simulink model "Dynamics"  (R2023a)
settings: Solver=FixedStepAuto  StartTime=0.0  StopTime=inf  FixedStep=0.001  EnableMultiTasking=on
libraries: sharedutil x32, sharedtransform x18, dspmtrx3 x12, matrix_library x6, simulink_extras x1, simulink x1
(part 2 of 6)

== system Dynamics/Subsystem/Z ==
  J(q) : Inport
  dq : Inport  Port=2
  Demux : Demux  Outputs=36
  Mux{,1..11} (12 alike) : Mux  Inputs=3
  Product : Product  Multiplication=Matrix(*)
  v1 : Outport
  v2 : Outport  Port=2
  v3 : Outport  Port=3
  v4 : Outport  Port=4
  v5 : Outport  Port=5
  v6 : Outport  Port=6
  w1 : Outport  Port=7
  w2 : Outport  Port=8
  w3 : Outport  Port=9
  w4 : Outport  Port=10
  w5 : Outport  Port=11
  w6 : Outport  Port=12
  Z : Outport  Port=13
  wires:
  J(q)/1 -> Product/1
  dq/1 -> Product/2
  Product/1 -> Z/1, Demux/1
  Demux/1 -> Mux/1
  Demux/2 -> Mux/2
  Demux/3 -> Mux/3
  Mux/1 -> v1/1
  Demux/4 -> Mux1/1
  Demux/5 -> Mux1/2
  Demux/6 -> Mux1/3
  Mux1/1 -> v2/1
  Mux2/1 -> v3/1
  Demux/7 -> Mux2/1
  Demux/8 -> Mux2/2
  Demux/9 -> Mux2/3
  Mux3/1 -> v4/1
  Demux/10 -> Mux3/1
  Demux/11 -> Mux3/2
  Demux/12 -> Mux3/3
  Mux4/1 -> v5/1
  Demux/14 -> Mux4/2
  Demux/13 -> Mux4/1
  Demux/15 -> Mux4/3
  Mux5/1 -> v6/1
  Demux/17 -> Mux5/2
  Demux/16 -> Mux5/1
  Demux/18 -> Mux5/3
  Mux6/1 -> w1/1
  Demux/19 -> Mux6/1
  Demux/20 -> Mux6/2
  Demux/21 -> Mux6/3
  Mux7/1 -> w2/1
  Demux/22 -> Mux7/1
  Demux/23 -> Mux7/2
  Demux/24 -> Mux7/3
  Mux8/1 -> w3/1
  Demux/25 -> Mux8/1
  Demux/26 -> Mux8/2
  Demux/27 -> Mux8/3
  Mux9/1 -> w4/1
  Demux/28 -> Mux9/1
  Demux/29 -> Mux9/2
  Demux/30 -> Mux9/3
  Mux10/1 -> w5/1
  Demux/31 -> Mux10/1
  Demux/32 -> Mux10/2
  Demux/33 -> Mux10/3
  Mux11/1 -> w6/1
  Demux/34 -> Mux11/1
  Demux/35 -> Mux11/2
  Demux/36 -> Mux11/3

== system Dynamics/Subsystem/tau(t) ==
  g(q) : Inport
  Add : Sum
  Constant : Constant  Value=zeros(5,1)
  Gain : Gain  Gain=0
  Mux : Mux  Inputs=2
  Sine Wave : Sin  SampleTime=0
  tau : Outport
  wires:
  Sine Wave/1 -> Mux/2
  Constant/1 -> Mux/1
  Add/1 -> tau/1
  Mux/1 -> Gain/1
  g(q)/1 -> Add/1
  Gain/1 -> Add/2

== system Dynamics/Subsystem2/Dynamics ==
  M(q) : Inport
  C(q,dq) : Inport  Port=2
  g(q) : Inport  Port=3
  dq : Inport  Port=4
  tau : Inport  Port=5
  q0 : Inport  Port=6
  dq0 : Inport  Port=7
  Add : Sum
  Add1 : Sum
  Gain : Gain  Gain=-1
  "Integrator, Second-Order" : SecondOrderIntegrator  ICSourceX=external  ICSourceDXDT=external
  Interpreted MATLAB Function : MATLABFcn  MATLABFcn=inv  OutputSignalType=real  Output1D=off
  Product : Product  Multiplication=Matrix(*)
  Product1 : Product  Multiplication=Matrix(*)
  q+delta_q : Outport
  dq+delta_dq : Outport  Port=2
  wires:
  C(q,dq)/1 -> Product/1
  dq/1 -> Product/2
  Product/1 -> Add/1
  g(q)/1 -> Add/2
  Add/1 -> Gain/1
  M(q)/1 -> Interpreted MATLAB Function/1
  Interpreted MATLAB Function/1 -> Product1/1
  Gain/1 -> Add1/1
  tau/1 -> Add1/2
  Add1/1 -> Product1/2
  Product1/1 -> "Integrator, Second-Order"/1
  "Integrator, Second-Order"/2 -> dq+delta_dq/1
  "Integrator, Second-Order"/1 -> q+delta_q/1
  q0/1 -> "Integrator, Second-Order"/2
  dq0/1 -> "Integrator, Second-Order"/3

== system Dynamics/Subsystem2/F gen. ==
  M : Inport
  H : Inport  Port=2
  G : Inport  Port=3
  Z : Inport  Port=4
  Add : Sum  Inputs=+++
  Derivative : Derivative
  Product1 : Product  Multiplication=Matrix(*)
  Product2 : Product  Multiplication=Matrix(*)
  F : Outport
  wires:
  Z/1 -> Product1/2, Derivative/1
  Add/1 -> F/1
  G/1 -> Add/3
  Product2/1 -> Add/1
  M/1 -> Product2/1
  Derivative/1 -> Product2/2
  Product1/1 -> Add/2
  H/1 -> Product1/1

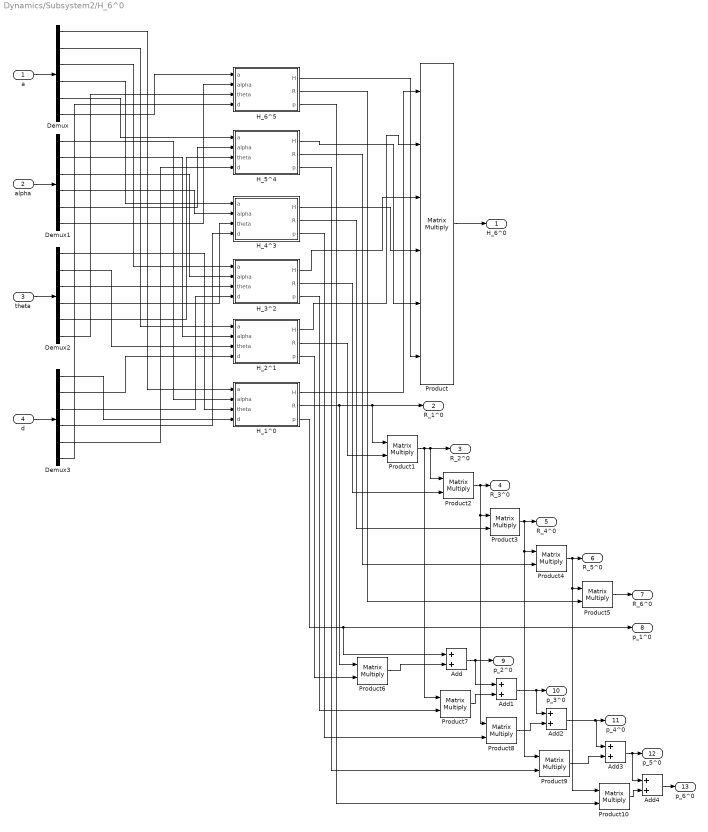
== system Dynamics/Subsystem2/H_6^0 ==
  a : Inport
  alpha : Inport  Port=2
  theta : Inport  Port=3
  d : Inport  Port=4
  Add{,1..4} (5 alike) : Sum
  Demux{,1..3} (4 alike) : Demux  Outputs=6
  H_1^0 : Subsystem
  H_2^1 : Subsystem
  H_3^2 : Subsystem
  H_4^3 : Subsystem
  H_5^4 : Subsystem
  H_6^5 : Subsystem
  Product : Product  Inputs=6  Multiplication=Matrix(*)
  Product{1..10} (10 alike) : Product  Multiplication=Matrix(*)
  H_6^0 : Outport
  R_1^0 : Outport  Port=2
  R_2^0 : Outport  Port=3
  R_3^0 : Outport  Port=4
  R_4^0 : Outport  Port=5
  R_5^0 : Outport  Port=6
  R_6^0 : Outport  Port=7
  p_1^0 : Outport  Port=8
  p_2^0 : Outport  Port=9
  p_3^0 : Outport  Port=10
  p_4^0 : Outport  Port=11
  p_5^0 : Outport  Port=12
  p_6^0 : Outport  Port=13
  wires:
  H_6^5/1(H) -> Product/6
  H_5^4/1(H) -> Product/5
  H_2^1/1(H) -> Product/2
  H_1^0/1(H) -> Product/1
  Product/1 -> H_6^0/1
  a/1 -> Demux/1
  d/1 -> Demux3/1
  H_4^3/1(H) -> Product/4
  H_3^2/1(H) -> Product/3
  Product1/1 -> Product7/1, Product2/1, R_2^0/1
  H_2^1/2(R) -> Product1/2
  Product2/1 -> Product8/1, Product3/1, R_3^0/1
  Product3/1 -> Product9/1, Product4/1, R_4^0/1
  Product4/1 -> Product10/1, Product5/1, R_5^0/1
  Product5/1 -> R_6^0/1
  Add/1 -> Add1/1, p_2^0/1
  theta/1 -> Demux2/1
  alpha/1 -> Demux1/1
  Demux/1 -> H_1^0/1(a)
  Demux/6 -> H_6^5/1(a)
  Demux/5 -> H_5^4/1(a)
  Demux/4 -> H_4^3/1(a)
  Demux/3 -> H_3^2/1(a)
  Demux/2 -> H_2^1/1(a)
  Demux1/6 -> H_6^5/2(alpha)
  Demux1/5 -> H_5^4/2(alpha)
  Demux1/4 -> H_4^3/2(alpha)
  Demux1/3 -> H_3^2/2(alpha)
  Demux1/2 -> H_2^1/2(alpha)
  Demux1/1 -> H_1^0/2(alpha)
  Demux2/6 -> H_6^5/3(theta)
  Demux2/5 -> H_5^4/3(theta)
  Demux2/4 -> H_4^3/3(theta)
  Demux2/3 -> H_3^2/3(theta)
  Demux2/2 -> H_2^1/3(theta)
  Demux2/1 -> H_1^0/3(theta)
  Demux3/1 -> H_1^0/4(d)
  Demux3/2 -> H_2^1/4(d)
  Demux3/3 -> H_3^2/4(d)
  Demux3/4 -> H_4^3/4(d)
  Demux3/5 -> H_5^4/4(d)
  Demux3/6 -> H_6^5/4(d)
  H_3^2/2(R) -> Product2/2
  H_4^3/2(R) -> Product3/2
  H_5^4/2(R) -> Product4/2
  H_6^5/2(R) -> Product5/2
  H_1^0/3(p) -> Add/1, p_1^0/1
  H_2^1/3(p) -> Product6/2
  Add1/1 -> Add2/1, p_3^0/1
  H_3^2/3(p) -> Product7/2
  H_4^3/3(p) -> Product8/2
  Add2/1 -> Add3/1, p_4^0/1
  H_5^4/3(p) -> Product9/2
  Add3/1 -> Add4/1, p_5^0/1
  H_6^5/3(p) -> Product10/2
  Add4/1 -> p_6^0/1
  H_1^0/2(R) -> R_1^0/1, Product1/1, Product6/1
  Product6/1 -> Add/2
  Product7/1 -> Add1/2
  Product8/1 -> Add2/2
  Product9/1 -> Add3/2
  Product10/1 -> Add4/2

== system Dynamics/Subsystem2/Jacobian ==
  R_1^0 : Inport
  R_2^0 : Inport  Port=2
  R_3^0 : Inport  Port=3
  R_4^0 : Inport  Port=4
  R_5^0 : Inport  Port=5
  R_6^0 : Inport  Port=6
  p_1^0 : Inport  Port=7
  p_2^0 : Inport  Port=8
  p_3^0 : Inport  Port=9
  p_4^0 : Inport  Port=10
  p_5^0 : Inport  Port=11
  p_6^0 : Inport  Port=12
  type1 : Inport  Port=13
  type2 : Inport  Port=14
  type3 : Inport  Port=15
  type4 : Inport  Port=16
  type5 : Inport  Port=17
  type6 : Inport  Port=18
  J(q) gen. : Subsystem
  J_v : Subsystem
  J_w : Subsystem
  Vector Concatenate : Concatenate  Mode=Multidimensional array
  J : Outport
  J(q) : Outport  Port=2
  wires:
  R_1^0/1 -> J_v/1(R_1^0), J_w/1(R_1^0), J(q) gen./1(R_1^0)
  p_1^0/1 -> J_v/7(p_1^0), J(q) gen./7(p_1^0)
  p_2^0/1 -> J_v/8(p_2^0), J(q) gen./8(p_2^0)
  p_3^0/1 -> J_v/9(p_3^0), J(q) gen./9(p_3^0)
  p_4^0/1 -> J_v/10(p_4^0), J(q) gen./10(p_4^0)
  p_5^0/1 -> J_v/11(p_5^0), J(q) gen./11(p_5^0)
  R_2^0/1 -> J_v/2(R_2^0), J_w/2(R_2^0), J(q) gen./2(R_2^0)
  R_3^0/1 -> J_v/3(R_3^0), J_w/3(R_3^0), J(q) gen./3(R_3^0)
  R_4^0/1 -> J_v/4(R_4^0), J_w/4(R_4^0), J(q) gen./4(R_4^0)
  R_5^0/1 -> J_v/5(R_5^0), J_w/5(R_5^0), J(q) gen./5(R_5^0)
  type1/1 -> J_w/7(type1), J_v/13(type1), J(q) gen./12(type1)
  type2/1 -> J_w/8(type2), J(q) gen./13(type2), J_v/14(type2)
  type3/1 -> J_w/9(type3), J(q) gen./14(type3), J_v/15(type3)
  type4/1 -> J_w/10(type4), J(q) gen./15(type4), J_v/16(type4)
  type5/1 -> J_w/11(type5), J_v/17(type5)
  type6/1 -> J_w/12(type6), J_v/18(type6)
  p_6^0/1 -> J_v/12(p_6^0)
  J_v/1(J_v) -> J(q) gen./16(J_v_6(q)), Vector Concatenate/1
  J_w/1(EF J_w) -> Vector Concatenate/2
  Vector Concatenate/1 -> J/1
  J(q) gen./1(J(q)) -> J(q)/1
  J_w/2(J_w1) -> J(q) gen./17(J_w1)
  J_w/3(J_w2) -> J(q) gen./18(J_w2)
  J_w/4(J_w3) -> J(q) gen./19(J_w3)
  J_w/5(J_w4) -> J(q) gen./20(J_w4)
  J_w/6(J_w5) -> J(q) gen./21(J_w5)
  J_w/7(J_w6) -> J(q) gen./22(J_w6)
  R_6^0/1 -> J_v/6(R_6^0), J_w/6(R_6^0), J(q) gen./6(R_6^0)

== system Dynamics/Subsystem2/M(q),C(q,dq),g(q) ==
  m : Inport
  J(q) : Inport  Port=2
  I1 : Inport  Port=3
  I2 : Inport  Port=4
  I3 : Inport  Port=5
  I4 : Inport  Port=6
  I5 : Inport  Port=7
  I6 : Inport  Port=8
  w1 : Inport  Port=9
  w2 : Inport  Port=10
  w3 : Inport  Port=11
  w4 : Inport  Port=12
  w5 : Inport  Port=13
  w6 : Inport  Port=14
  Add : Sum
  G gen : Subsystem
  Interpreted MATLAB Function : MATLABFcn  MATLABFcn=transpose  OutputSignalType=real  Output1D=off
  M,H : Subsystem
  Product{,1..3} (4 alike) : Product  Multiplication=Matrix(*)
  Product4 : Product  Inputs=3  Multiplication=Matrix(*)
  dJ : Derivative
  g(q) : Outport
  C(q,dq) : Outport  Port=2
  M(q) : Outport  Port=3
  M : Outport  Port=4
  H : Outport  Port=5
  G : Outport  Port=6
  wires:
  J(q)/1 -> Interpreted MATLAB Function/1, Product4/3, Product2/2, dJ/1
  Interpreted MATLAB Function/1 -> Product4/1, Product3/1, Product/1
  Product/1 -> g(q)/1
  m/1 -> G gen/1(m), M,H/1(m)
  I1/1 -> M,H/2(I1)
  I2/1 -> M,H/3(I2)
  I3/1 -> M,H/4(I3)
  I4/1 -> M,H/5(I4)
  I5/1 -> M,H/6(I5)
  I6/1 -> M,H/7(I6)
  w1/1 -> M,H/8(w1)
  w2/1 -> M,H/9(w2)
  w3/1 -> M,H/10(w3)
  w4/1 -> M,H/11(w4)
  w5/1 -> M,H/12(w5)
  w6/1 -> M,H/13(w6)
  M,H/1(M) -> Product1/1, M/1, Product4/2
  dJ/1 -> Product1/2
  M,H/2(H) -> H/1, Product2/1
  Product1/1 -> Add/1
  Product2/1 -> Add/2
  Add/1 -> Product3/2
  Product3/1 -> C(q,dq)/1
  Product4/1 -> M(q)/1
  G gen/1(G) -> G/1, Product/2

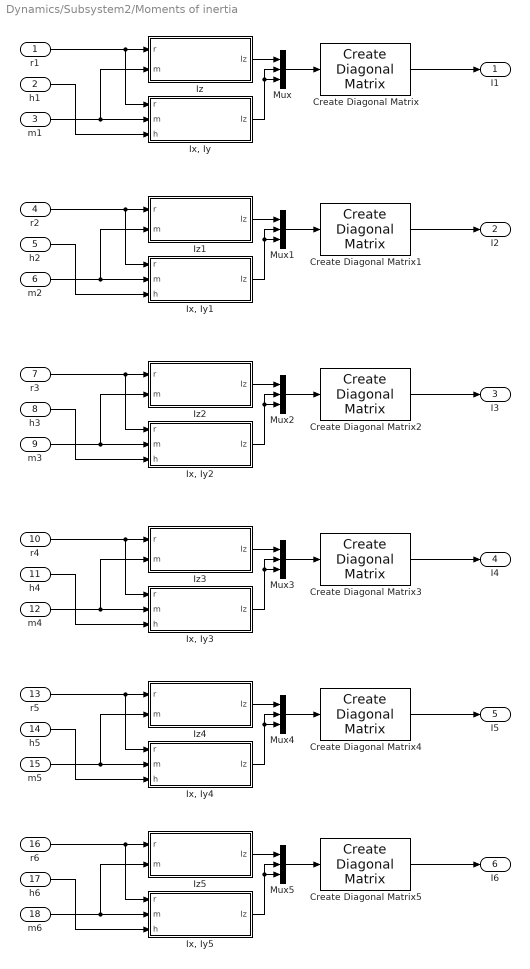
== system Dynamics/Subsystem2/Moments of inertia ==
  r1 : Inport
  h1 : Inport  Port=2
  m1 : Inport  Port=3
  r2 : Inport  Port=4
  h2 : Inport  Port=5
  m2 : Inport  Port=6
  r3 : Inport  Port=7
  h3 : Inport  Port=8
  m3 : Inport  Port=9
  r4 : Inport  Port=10
  h4 : Inport  Port=11
  m4 : Inport  Port=12
  r5 : Inport  Port=13
  h5 : Inport  Port=14
  m5 : Inport  Port=15
  r6 : Inport  Port=16
  h6 : Inport  Port=17
  m6 : Inport  Port=18
  Create Diagonal Matrix{,1..5} (6 alike) : matrix_library/Create Diagonal Matrix
  "Ix, Iy" : Subsystem
  "Ix, Iy1" : Subsystem
  "Ix, Iy2" : Subsystem
  "Ix, Iy3" : Subsystem
  "Ix, Iy4" : Subsystem
  "Ix, Iy5" : Subsystem
  Iz : Subsystem
  Iz1 : Subsystem
  Iz2 : Subsystem
  Iz3 : Subsystem
  Iz4 : Subsystem
  Iz5 : Subsystem
  Mux{,1..5} (6 alike) : Mux  Inputs=3
  I1 : Outport
  I2 : Outport  Port=2
  I3 : Outport  Port=3
  I4 : Outport  Port=4
  I5 : Outport  Port=5
  I6 : Outport  Port=6
  wires:
  r1/1 -> "Ix, Iy"/1(r), Iz/1(r)
  m1/1 -> "Ix, Iy"/2(m), Iz/2(m)
  h1/1 -> "Ix, Iy"/3(h)
  Mux/1 -> Create Diagonal Matrix/1
  Iz/1(Iz) -> Mux/1
  "Ix, Iy"/1(Iz) -> Mux/3, Mux/2
  Create Diagonal Matrix/1 -> I1/1
  r2/1 -> "Ix, Iy1"/1(r), Iz1/1(r)
  m2/1 -> "Ix, Iy1"/2(m), Iz1/2(m)
  h2/1 -> "Ix, Iy1"/3(h)
  Mux1/1 -> Create Diagonal Matrix1/1
  Iz1/1(Iz) -> Mux1/1
  "Ix, Iy1"/1(Iz) -> Mux1/3, Mux1/2
  Create Diagonal Matrix1/1 -> I2/1
  r3/1 -> "Ix, Iy2"/1(r), Iz2/1(r)
  m3/1 -> "Ix, Iy2"/2(m), Iz2/2(m)
  h3/1 -> "Ix, Iy2"/3(h)
  Mux2/1 -> Create Diagonal Matrix2/1
  Iz2/1(Iz) -> Mux2/1
  "Ix, Iy2"/1(Iz) -> Mux2/3, Mux2/2
  Create Diagonal Matrix2/1 -> I3/1
  r4/1 -> "Ix, Iy3"/1(r), Iz3/1(r)
  m4/1 -> "Ix, Iy3"/2(m), Iz3/2(m)
  h4/1 -> "Ix, Iy3"/3(h)
  Mux3/1 -> Create Diagonal Matrix3/1
  Iz3/1(Iz) -> Mux3/1
  "Ix, Iy3"/1(Iz) -> Mux3/3, Mux3/2
  Create Diagonal Matrix3/1 -> I4/1
  r5/1 -> "Ix, Iy4"/1(r), Iz4/1(r)
  m5/1 -> "Ix, Iy4"/2(m), Iz4/2(m)
  h5/1 -> "Ix, Iy4"/3(h)
  Mux4/1 -> Create Diagonal Matrix4/1
  Iz4/1(Iz) -> Mux4/1
  "Ix, Iy4"/1(Iz) -> Mux4/3, Mux4/2
  Create Diagonal Matrix4/1 -> I5/1
  r6/1 -> "Ix, Iy5"/1(r), Iz5/1(r)
  m6/1 -> "Ix, Iy5"/2(m), Iz5/2(m)
  h6/1 -> "Ix, Iy5"/3(h)
  Mux5/1 -> Create Diagonal Matrix5/1
  Iz5/1(Iz) -> Mux5/1
  "Ix, Iy5"/1(Iz) -> Mux5/3, Mux5/2
  Create Diagonal Matrix5/1 -> I6/1

== system Dynamics/Subsystem2/Slotine ==
  g(q) : Inport
  C(q,dq) : Inport  Port=2
  M(q) : Inport  Port=3
  q_d : Inport  Port=4
  dq_d : Inport  Port=5
  ddq_d : Inport  Port=6
  q : Inport  Port=7
  dq : Inport  Port=8
  Lambda : Inport  Port=9
  K : Inport  Port=10
  S-gen : Subsystem
  V-gen : Subsystem
  dV-gen : Subsystem
  dq_tilde : Sum  Inputs=-+
  q_tilde : Sum  Inputs=-+
  tau-gen : Subsystem
  tau : Outport
  wires:
  q_d/1 -> q_tilde/1
  q/1 -> q_tilde/2
  dq_d/1 -> V-gen/2(dq_d), dq_tilde/1
  dq/1 -> S-gen/1(dq), dq_tilde/2
  ddq_d/1 -> dV-gen/2(ddq_d)
  q_tilde/1 -> V-gen/1(q_tilde)
  Lambda/1 -> dV-gen/3(Gamma), V-gen/3(Gamma)
  dq_tilde/1 -> dV-gen/1(dq_tilde)
  V-gen/1(V) -> tau-gen/4(V), S-gen/2(V)
  M(q)/1 -> tau-gen/1(M)
  C(q,dq)/1 -> tau-gen/2(C)
  g(q)/1 -> tau-gen/3(g)
  dV-gen/1(dV) -> tau-gen/5(dV)
  S-gen/1(S) -> tau-gen/6(S)
  K/1 -> tau-gen/7(K)
  tau-gen/1(tau) -> tau/1

== system Dynamics/Subsystem2/Z ==
  J(q) : Inport
  dq : Inport  Port=2
  Demux : Demux  Outputs=36
  Mux{,1..11} (12 alike) : Mux  Inputs=3
  Product : Product  Multiplication=Matrix(*)
  v1 : Outport
  v2 : Outport  Port=2
  v3 : Outport  Port=3
  v4 : Outport  Port=4
  v5 : Outport  Port=5
  v6 : Outport  Port=6
  w1 : Outport  Port=7
  w2 : Outport  Port=8
  w3 : Outport  Port=9
  w4 : Outport  Port=10
  w5 : Outport  Port=11
  w6 : Outport  Port=12
  Z : Outport  Port=13
  wires:
  J(q)/1 -> Product/1
  dq/1 -> Product/2
  Product/1 -> Z/1, Demux/1
  Demux/1 -> Mux/1
  Demux/2 -> Mux/2
  Demux/3 -> Mux/3
  Mux/1 -> v1/1
  Demux/4 -> Mux1/1
  Demux/5 -> Mux1/2
  Demux/6 -> Mux1/3
  Mux1/1 -> v2/1
  Mux2/1 -> v3/1
  Demux/7 -> Mux2/1
  Demux/8 -> Mux2/2
  Demux/9 -> Mux2/3
  Mux3/1 -> v4/1
  Demux/10 -> Mux3/1
  Demux/11 -> Mux3/2
  Demux/12 -> Mux3/3
  Mux4/1 -> v5/1
  Demux/14 -> Mux4/2
  Demux/13 -> Mux4/1
  Demux/15 -> Mux4/3
  Mux5/1 -> v6/1
  Demux/17 -> Mux5/2
  Demux/16 -> Mux5/1
  Demux/18 -> Mux5/3
  Mux6/1 -> w1/1
  Demux/19 -> Mux6/1
  Demux/20 -> Mux6/2
  Demux/21 -> Mux6/3
  Mux7/1 -> w2/1
  Demux/22 -> Mux7/1
  Demux/23 -> Mux7/2
  Demux/24 -> Mux7/3
  Mux8/1 -> w3/1
  Demux/25 -> Mux8/1
  Demux/26 -> Mux8/2
  Demux/27 -> Mux8/3
  Mux9/1 -> w4/1
  Demux/28 -> Mux9/1
  Demux/29 -> Mux9/2
  Demux/30 -> Mux9/3
  Mux10/1 -> w5/1
  Demux/31 -> Mux10/1
  Demux/32 -> Mux10/2
  Demux/33 -> Mux10/3
  Mux11/1 -> w6/1
  Demux/34 -> Mux11/1
  Demux/35 -> Mux11/2
  Demux/36 -> Mux11/3

== system Dynamics/Subsystem2/tau(t) ==
  g(q) : Inport
  Add : Sum
  Constant : Constant  Value=zeros(5,1)
  Gain : Gain  Gain=0
  Mux : Mux  Inputs=2
  Sine Wave : Sin  SampleTime=0
  tau : Outport
  wires:
  Sine Wave/1 -> Mux/2
  Constant/1 -> Mux/1
  Add/1 -> tau/1
  Mux/1 -> Gain/1
  g(q)/1 -> Add/1
  Gain/1 -> Add/2

== system Dynamics/DYNAMIC/H_6^0/H_1^0 ==
  a : Inport
  alpha : Inport  Port=2
  theta : Inport  Port=3
  d : Inport  Port=4
  Gain1 : Gain  Gain=-1
  Gain2 : Gain  Gain=-1
  MATLAB Function : MATLAB Function  TreatAsAtomicUnit=on
  Mux : Mux  Inputs=3
  Mux1 : Mux  Inputs=3
  Product : Product
  Product1 : Product
  Rotation Angles to Direction Cosine Matrix : sharedtransform/Rotation Angles to Direction Cosine Matrix  rotationOrder=ZXY  aMode=aMode
  Trigonometric Function : Trigonometry  Operator=cos
  Trigonometric Function1 : Trigonometry
  Zero : Constant  Value=0
  H : Outport
  R : Outport  Port=2
  p : Outport  Port=3
  wires:
  Mux/1 -> Rotation Angles to Direction Cosine Matrix/1
  alpha/1 -> Gain1/1
  Zero/1 -> Mux/3
  Rotation Angles to Direction Cosine Matrix/1 -> MATLAB Function/1(R), R/1
  Mux1/1 -> MATLAB Function/2(p), p/1
  Trigonometric Function/1 -> Product/1
  Trigonometric Function1/1 -> Product1/1
  Product/1 -> Mux1/1
  Product1/1 -> Mux1/2
  a/1 -> Product/2, Product1/2
  MATLAB Function/1(H) -> H/1
  Gain1/1 -> Mux/1
  Gain2/1 -> Mux/2
  theta/1 -> Trigonometric Function1/1, Trigonometric Function/1, Gain2/1
  d/1 -> Mux1/3

== system Dynamics/DYNAMIC/H_6^0/H_2^1 ==
  a : Inport
  alpha : Inport  Port=2
  theta : Inport  Port=3
  d : Inport  Port=4
  Gain1 : Gain  Gain=-1
  Gain2 : Gain  Gain=-1
  MATLAB Function : MATLAB Function  TreatAsAtomicUnit=on
  Mux : Mux  Inputs=3
  Mux1 : Mux  Inputs=3
  Product : Product
  Product1 : Product
  Rotation Angles to Direction Cosine Matrix : sharedtransform/Rotation Angles to Direction Cosine Matrix  rotationOrder=ZXY  aMode=aMode
  Trigonometric Function : Trigonometry  Operator=cos
  Trigonometric Function1 : Trigonometry
  Zero : Constant  Value=0
  H : Outport
  R : Outport  Port=2
  p : Outport  Port=3
  wires:
  Mux/1 -> Rotation Angles to Direction Cosine Matrix/1
  alpha/1 -> Gain1/1
  Zero/1 -> Mux/3
  Rotation Angles to Direction Cosine Matrix/1 -> MATLAB Function/1(R), R/1
  Mux1/1 -> MATLAB Function/2(p), p/1
  Trigonometric Function/1 -> Product/1
  Trigonometric Function1/1 -> Product1/1
  Product/1 -> Mux1/1
  Product1/1 -> Mux1/2
  a/1 -> Product/2, Product1/2
  MATLAB Function/1(H) -> H/1
  Gain1/1 -> Mux/1
  Gain2/1 -> Mux/2
  theta/1 -> Trigonometric Function1/1, Trigonometric Function/1, Gain2/1
  d/1 -> Mux1/3

== system Dynamics/DYNAMIC/H_6^0/H_3^2 ==
  a : Inport
  alpha : Inport  Port=2
  theta : Inport  Port=3
  d : Inport  Port=4
  Gain1 : Gain  Gain=-1
  Gain2 : Gain  Gain=-1
  MATLAB Function : MATLAB Function  TreatAsAtomicUnit=on
  Mux : Mux  Inputs=3
  Mux1 : Mux  Inputs=3
  Product : Product
  Product1 : Product
  Rotation Angles to Direction Cosine Matrix : sharedtransform/Rotation Angles to Direction Cosine Matrix  rotationOrder=ZXY  aMode=aMode
  Trigonometric Function : Trigonometry  Operator=cos
  Trigonometric Function1 : Trigonometry
  Zero : Constant  Value=0
  H : Outport
  R : Outport  Port=2
  p : Outport  Port=3
  wires:
  Mux/1 -> Rotation Angles to Direction Cosine Matrix/1
  alpha/1 -> Gain1/1
  Zero/1 -> Mux/3
  Rotation Angles to Direction Cosine Matrix/1 -> MATLAB Function/1(R), R/1
  Mux1/1 -> MATLAB Function/2(p), p/1
  Trigonometric Function/1 -> Product/1
  Trigonometric Function1/1 -> Product1/1
  Product/1 -> Mux1/1
  Product1/1 -> Mux1/2
  a/1 -> Product/2, Product1/2
  MATLAB Function/1(H) -> H/1
  Gain1/1 -> Mux/1
  Gain2/1 -> Mux/2
  theta/1 -> Trigonometric Function1/1, Trigonometric Function/1, Gain2/1
  d/1 -> Mux1/3

== system Dynamics/DYNAMIC/H_6^0/H_4^3 ==
  a : Inport
  alpha : Inport  Port=2
  theta : Inport  Port=3
  d : Inport  Port=4
  Gain1 : Gain  Gain=-1
  Gain2 : Gain  Gain=-1
  MATLAB Function : MATLAB Function  TreatAsAtomicUnit=on
  Mux : Mux  Inputs=3
  Mux1 : Mux  Inputs=3
  Product : Product
  Product1 : Product
  Rotation Angles to Direction Cosine Matrix : sharedtransform/Rotation Angles to Direction Cosine Matrix  rotationOrder=ZXY  aMode=aMode
  Trigonometric Function : Trigonometry  Operator=cos
  Trigonometric Function1 : Trigonometry
  Zero : Constant  Value=0
  H : Outport
  R : Outport  Port=2
  p : Outport  Port=3
  wires:
  Mux/1 -> Rotation Angles to Direction Cosine Matrix/1
  alpha/1 -> Gain1/1
  Zero/1 -> Mux/3
  Rotation Angles to Direction Cosine Matrix/1 -> MATLAB Function/1(R), R/1
  Mux1/1 -> MATLAB Function/2(p), p/1
  Trigonometric Function/1 -> Product/1
  Trigonometric Function1/1 -> Product1/1
  Product/1 -> Mux1/1
  Product1/1 -> Mux1/2
  a/1 -> Product/2, Product1/2
  MATLAB Function/1(H) -> H/1
  Gain1/1 -> Mux/1
  Gain2/1 -> Mux/2
  theta/1 -> Trigonometric Function1/1, Trigonometric Function/1, Gain2/1
  d/1 -> Mux1/3

== system Dynamics/DYNAMIC/H_6^0/H_5^4 ==
  a : Inport
  alpha : Inport  Port=2
  theta : Inport  Port=3
  d : Inport  Port=4
  Gain1 : Gain  Gain=-1
  Gain2 : Gain  Gain=-1
  MATLAB Function : MATLAB Function  TreatAsAtomicUnit=on
  Mux : Mux  Inputs=3
  Mux1 : Mux  Inputs=3
  Product : Product
  Product1 : Product
  Rotation Angles to Direction Cosine Matrix : sharedtransform/Rotation Angles to Direction Cosine Matrix  rotationOrder=ZXY  aMode=aMode
  Trigonometric Function : Trigonometry  Operator=cos
  Trigonometric Function1 : Trigonometry
  Zero : Constant  Value=0
  H : Outport
  R : Outport  Port=2
  p : Outport  Port=3
  wires:
  Mux/1 -> Rotation Angles to Direction Cosine Matrix/1
  alpha/1 -> Gain1/1
  Zero/1 -> Mux/3
  Rotation Angles to Direction Cosine Matrix/1 -> MATLAB Function/1(R), R/1
  Mux1/1 -> MATLAB Function/2(p), p/1
  Trigonometric Function/1 -> Product/1
  Trigonometric Function1/1 -> Product1/1
  Product/1 -> Mux1/1
  Product1/1 -> Mux1/2
  a/1 -> Product/2, Product1/2
  MATLAB Function/1(H) -> H/1
  Gain1/1 -> Mux/1
  Gain2/1 -> Mux/2
  theta/1 -> Trigonometric Function1/1, Trigonometric Function/1, Gain2/1
  d/1 -> Mux1/3

== system Dynamics/DYNAMIC/H_6^0/H_6^5 ==
  a : Inport
  alpha : Inport  Port=2
  theta : Inport  Port=3
  d : Inport  Port=4
  Gain1 : Gain  Gain=-1
  Gain2 : Gain  Gain=-1
  MATLAB Function : MATLAB Function  TreatAsAtomicUnit=on
  Mux : Mux  Inputs=3
  Mux1 : Mux  Inputs=3
  Product : Product
  Product1 : Product
  Rotation Angles to Direction Cosine Matrix : sharedtransform/Rotation Angles to Direction Cosine Matrix  rotationOrder=ZXY  aMode=aMode
  Trigonometric Function : Trigonometry  Operator=cos
  Trigonometric Function1 : Trigonometry
  Zero : Constant  Value=0
  H : Outport
  R : Outport  Port=2
  p : Outport  Port=3
  wires:
  Mux/1 -> Rotation Angles to Direction Cosine Matrix/1
  alpha/1 -> Gain1/1
  Zero/1 -> Mux/3
  Rotation Angles to Direction Cosine Matrix/1 -> MATLAB Function/1(R), R/1
  Mux1/1 -> MATLAB Function/2(p), p/1
  Trigonometric Function/1 -> Product/1
  Trigonometric Function1/1 -> Product1/1
  Product/1 -> Mux1/1
  Product1/1 -> Mux1/2
  a/1 -> Product/2, Product1/2
  MATLAB Function/1(H) -> H/1
  Gain1/1 -> Mux/1
  Gain2/1 -> Mux/2
  theta/1 -> Trigonometric Function1/1, Trigonometric Function/1, Gain2/1
  d/1 -> Mux1/3

== system Dynamics/DYNAMIC/Jacobian/J(q) gen. ==
  R_1^0 : Inport
  R_2^0 : Inport  Port=2
  R_3^0 : Inport  Port=3
  R_4^0 : Inport  Port=4
  R_5^0 : Inport  Port=5
  R_6^0 : Inport  Port=6
  p_1^0 : Inport  Port=7
  p_2^0 : Inport  Port=8
  p_3^0 : Inport  Port=9
  p_4^0 : Inport  Port=10
  p_5^0 : Inport  Port=11
  type1 : Inport  Port=12
  type2 : Inport  Port=13
  type3 : Inport  Port=14
  type4 : Inport  Port=15
  J_v_6(q) : Inport  Port=16
  J_w1 : Inport  Port=17
  J_w2 : Inport  Port=18
  J_w3 : Inport  Port=19
  J_w4 : Inport  Port=20
  J_w5 : Inport  Port=21
  J_w6 : Inport  Port=22
  J_v_1(q) : Subsystem
  J_v_2(q) : Subsystem
  J_v_3(q) : Subsystem
  J_v_4(q) : Subsystem
  J_v_5(q) : Subsystem
  MATLAB Function : MATLAB Function  TreatAsAtomicUnit=on
  J(q) : Outport
  wires:
  MATLAB Function/1(J_q) -> J(q)/1
  J_v_6(q)/1 -> MATLAB Function/12(J_v6)
  J_w1/1 -> MATLAB Function/1(J_w1)
  J_w2/1 -> MATLAB Function/2(J_w2)
  J_w3/1 -> MATLAB Function/3(J_w3)
  J_w4/1 -> MATLAB Function/4(J_w4)
  J_w5/1 -> MATLAB Function/5(J_w5)
  J_w6/1 -> MATLAB Function/6(J_w6)
  J_v_1(q)/1(J_v_1(q)) -> MATLAB Function/7(J_v1)
  J_v_2(q)/1(J_v_2(q)) -> MATLAB Function/8(J_v2)
  J_v_3(q)/1(J_v_3(q)) -> MATLAB Function/9(J_v3)
  J_v_4(q)/1(J_v_4(q)) -> MATLAB Function/10(J_v4)
  J_v_5(q)/1(J_v_5(q)) -> MATLAB Function/11(J_v5)
  R_5^0/1 -> MATLAB Function/17(R5)
  R_6^0/1 -> MATLAB Function/18(R6)
  R_1^0/1 -> MATLAB Function/13(R1), J_v_5(q)/1(R_1^0), J_v_4(q)/1(R_1^0), J_v_3(q)/1(R_1^0), J_v_2(q)/1(R_1^0)
  R_2^0/1 -> MATLAB Function/14(R2), J_v_5(q)/2(R_2^0), J_v_4(q)/2(R_2^0), J_v_3(q)/2(R_2^0)
  R_3^0/1 -> J_v_4(q)/3(R_3^0), MATLAB Function/15(R3), J_v_5(q)/3(R_3^0)
  R_4^0/1 -> MATLAB Function/16(R4), J_v_5(q)/4(R_4^0)
  p_1^0/1 -> J_v_5(q)/5(p_1^0), J_v_4(q)/4(p_1^0), J_v_3(q)/3(p_1^0), J_v_2(q)/2(p_1^0)
  p_2^0/1 -> J_v_5(q)/6(p_2^0), J_v_4(q)/5(p_2^0), J_v_3(q)/4(p_2^0), J_v_2(q)/3(p_2^0)
  p_3^0/1 -> J_v_3(q)/5(p_3^0), J_v_5(q)/7(p_3^0), J_v_4(q)/6(p_3^0)
  p_4^0/1 -> J_v_5(q)/8(p_4^0), J_v_4(q)/7(p_4^0)
  p_5^0/1 -> J_v_5(q)/9(p_5^0)
  type1/1 -> J_v_5(q)/10(type1), J_v_4(q)/8(type1), J_v_3(q)/6(type1), J_v_2(q)/4(type1)
  type2/1 -> J_v_5(q)/11(type2), J_v_4(q)/9(type2), J_v_3(q)/7(type2)
  type3/1 -> J_v_5(q)/12(type3), J_v_4(q)/10(type3)
  type4/1 -> J_v_5(q)/13(type4)

== system Dynamics/DYNAMIC/Jacobian/J_v ==
  R_1^0 : Inport
  R_2^0 : Inport  Port=2
  R_3^0 : Inport  Port=3
  R_4^0 : Inport  Port=4
  R_5^0 : Inport  Port=5
  R_6^0 : Inport  Port=6
  p_1^0 : Inport  Port=7
  p_2^0 : Inport  Port=8
  p_3^0 : Inport  Port=9
  p_4^0 : Inport  Port=10
  p_5^0 : Inport  Port=11
  p_6^0 : Inport  Port=12
  type1 : Inport  Port=13
  type2 : Inport  Port=14
  type3 : Inport  Port=15
  type4 : Inport  Port=16
  type5 : Inport  Port=17
  type6 : Inport  Port=18
  J_v_1 : Subsystem
  J_v_2 : Subsystem
  J_v_3 : Subsystem
  J_v_4 : Subsystem
  J_v_5 : Subsystem
  J_v_6 : Subsystem
  v2M_1 : MATLAB Function  TreatAsAtomicUnit=on
  v2M_2 : MATLAB Function  TreatAsAtomicUnit=on
  v2M_3 : MATLAB Function  TreatAsAtomicUnit=on
  v2M_4 : MATLAB Function  TreatAsAtomicUnit=on
  v2M_5 : MATLAB Function  TreatAsAtomicUnit=on
  J_v : Outport
  wires:
  R_1^0/1 -> J_v_1/1(R)
  J_v_1/1(J_v) -> v2M_1/1(v1)
  v2M_1/1(M) -> v2M_2/1(v1)
  v2M_2/1(M) -> v2M_3/1(v1)
  v2M_3/1(M) -> v2M_4/1(v1)
  v2M_4/1(M) -> v2M_5/1(v1)
  v2M_5/1(M) -> J_v/1
  J_v_2/1(J_v) -> v2M_1/2(v2)
  J_v_3/1(J_v) -> v2M_2/2(v2)
  J_v_4/1(J_v) -> v2M_3/2(v2)
  J_v_5/1(J_v) -> v2M_4/2(v2)
  J_v_6/1(J_v) -> v2M_5/2(v2)
  R_2^0/1 -> J_v_2/1(R)
  R_3^0/1 -> J_v_3/1(R)
  R_4^0/1 -> J_v_4/1(R)
  R_5^0/1 -> J_v_5/1(R)
  R_6^0/1 -> J_v_6/1(R)
  p_1^0/1 -> J_v_1/2(p)
  p_2^0/1 -> J_v_2/2(p)
  p_3^0/1 -> J_v_3/2(p)
  p_4^0/1 -> J_v_4/2(p)
  p_5^0/1 -> J_v_5/2(p)
  type2/1 -> J_v_2/4(type)
  type1/1 -> J_v_1/4(type)
  type3/1 -> J_v_3/4(type)
  type4/1 -> J_v_4/4(type)
  type5/1 -> J_v_5/4(type)
  type6/1 -> J_v_6/4(type)
  p_6^0/1 -> J_v_6/2(p), J_v_1/3(pn), J_v_2/3(pn), J_v_3/3(pn), J_v_4/3(pn), J_v_5/3(pn), J_v_6/3(pn)

== system Dynamics/DYNAMIC/Jacobian/J_w ==
  R_1^0 : Inport
  R_2^0 : Inport  Port=2
  R_3^0 : Inport  Port=3
  R_4^0 : Inport  Port=4
  R_5^0 : Inport  Port=5
  R_6^0 : Inport  Port=6
  type1 : Inport  Port=7
  type2 : Inport  Port=8
  type3 : Inport  Port=9
  type4 : Inport  Port=10
  type5 : Inport  Port=11
  type6 : Inport  Port=12
  J_w_1 : MATLAB Function  TreatAsAtomicUnit=on
  J_w_2 : MATLAB Function  TreatAsAtomicUnit=on
  J_w_3 : MATLAB Function  TreatAsAtomicUnit=on
  J_w_4 : MATLAB Function  TreatAsAtomicUnit=on
  J_w_5 : MATLAB Function  TreatAsAtomicUnit=on
  J_w_6 : MATLAB Function  TreatAsAtomicUnit=on
  v2M_1 : MATLAB Function  TreatAsAtomicUnit=on
  v2M_2 : MATLAB Function  TreatAsAtomicUnit=on
  v2M_3 : MATLAB Function  TreatAsAtomicUnit=on
  v2M_4 : MATLAB Function  TreatAsAtomicUnit=on
  v2M_5 : MATLAB Function  TreatAsAtomicUnit=on
  EF J_w : Outport
  J_w1 : Outport  Port=2
  J_w2 : Outport  Port=3
  J_w3 : Outport  Port=4
  J_w4 : Outport  Port=5
  J_w5 : Outport  Port=6
  J_w6 : Outport  Port=7
  wires:
  R_1^0/1 -> J_w_1/1(R)
  R_2^0/1 -> J_w_2/1(R)
  R_3^0/1 -> J_w_3/1(R)
  R_4^0/1 -> J_w_4/1(R)
  R_5^0/1 -> J_w_5/1(R)
  R_6^0/1 -> J_w_6/1(R)
  J_w_1/1(J_w) -> J_w1/1, v2M_1/1(v1)
  J_w_2/1(J_w) -> J_w2/1, v2M_1/2(v2)
  J_w_3/1(J_w) -> J_w3/1, v2M_2/2(v2)
  v2M_1/1(M) -> v2M_2/1(v1)
  v2M_2/1(M) -> v2M_3/1(v1)
  v2M_3/1(M) -> v2M_4/1(v1)
  J_w_5/1(J_w) -> J_w5/1, v2M_4/2(v2)
  J_w_6/1(J_w) -> J_w6/1, v2M_5/2(v2)
  v2M_4/1(M) -> v2M_5/1(v1)
  v2M_5/1(M) -> EF J_w/1
  type1/1 -> J_w_1/2(type)
  type2/1 -> J_w_2/2(type)
  type3/1 -> J_w_3/2(type)
  type4/1 -> J_w_4/2(type)
  type5/1 -> J_w_5/2(type)
  type6/1 -> J_w_6/2(type)
  J_w_4/1(J_w) -> v2M_3/2(v2), J_w4/1

== system Dynamics/DYNAMIC/M(q),C(q,dq),g(q)/G gen ==
  m : Inport
  Demux : Demux  Outputs=6
  Mux : Mux  Inputs=7
  Product{,1..5} (6 alike) : Product
  g : Constant  Value=[0;0;9.81]
  g1 : Constant  Value=zeros(18,1)
  G : Outport
  wires:
  m/1 -> Demux/1
  Demux/1 -> Product/1
  Demux/2 -> Product1/1
  Demux/3 -> Product2/1
  g/1 -> Product5/2, Product4/2, Product3/2, Product2/2, Product1/2, Product/2
  Demux/4 -> Product3/1
  Demux/5 -> Product4/1
  Demux/6 -> Product5/1
  Product1/1 -> Mux/2
  Product/1 -> Mux/1
  Product2/1 -> Mux/3
  Product4/1 -> Mux/5
  Product5/1 -> Mux/6
  Product3/1 -> Mux/4
  g1/1 -> Mux/7
  Mux/1 -> G/1

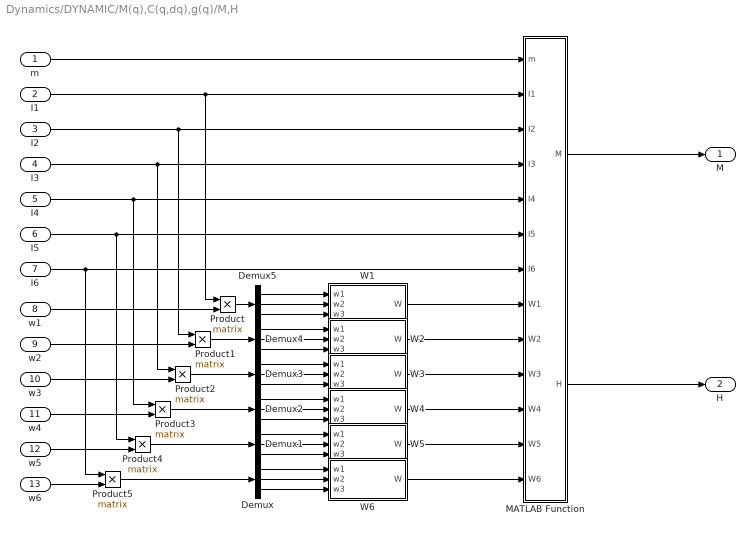
== system Dynamics/DYNAMIC/M(q),C(q,dq),g(q)/M,H ==
  m : Inport
  I1 : Inport  Port=2
  I2 : Inport  Port=3
  I3 : Inport  Port=4
  I4 : Inport  Port=5
  I5 : Inport  Port=6
  I6 : Inport  Port=7
  w1 : Inport  Port=8
  w2 : Inport  Port=9
  w3 : Inport  Port=10
  w4 : Inport  Port=11
  w5 : Inport  Port=12
  w6 : Inport  Port=13
  Demux{,1..5} (6 alike) : Demux  Outputs=3
  MATLAB Function : MATLAB Function  TreatAsAtomicUnit=on
  Product{,1..5} (6 alike) : Product  Multiplication=Matrix(*)
  W1 : MATLAB Function  TreatAsAtomicUnit=on
  W2 : MATLAB Function  TreatAsAtomicUnit=on
  W3 : MATLAB Function  TreatAsAtomicUnit=on
  W4 : MATLAB Function  TreatAsAtomicUnit=on
  W5 : MATLAB Function  TreatAsAtomicUnit=on
  W6 : MATLAB Function  TreatAsAtomicUnit=on
  M : Outport
  H : Outport  Port=2
  wires:
  m/1 -> MATLAB Function/1(m)
  I1/1 -> Product/1, MATLAB Function/2(I1)
  I2/1 -> Product1/1, MATLAB Function/3(I2)
  I3/1 -> Product2/1, MATLAB Function/4(I3)
  I4/1 -> Product3/1, MATLAB Function/5(I4)
  I5/1 -> Product4/1, MATLAB Function/6(I5)
  I6/1 -> Product5/1, MATLAB Function/7(I6)
  MATLAB Function/1(M) -> M/1
  MATLAB Function/2(H) -> H/1
  W1/1(W) -> MATLAB Function/8(W1)
  W2/1(W) -> MATLAB Function/9(W2)
  W3/1(W) -> MATLAB Function/10(W3)
  W4/1(W) -> MATLAB Function/11(W4)
  W5/1(W) -> MATLAB Function/12(W5)
  W6/1(W) -> MATLAB Function/13(W6)
  w6/1 -> Product5/2
  Demux/3 -> W6/3(w3)
  Demux/2 -> W6/2(w2)
  Demux/1 -> W6/1(w1)
  w5/1 -> Product4/2
  Demux1/3 -> W5/3(w3)
  Demux1/2 -> W5/2(w2)
  Demux1/1 -> W5/1(w1)
  w4/1 -> Product3/2
  Demux2/3 -> W4/3(w3)
  Demux2/2 -> W4/2(w2)
  Demux2/1 -> W4/1(w1)
  w3/1 -> Product2/2
  Demux3/3 -> W3/3(w3)
  Demux3/2 -> W3/2(w2)
  Demux3/1 -> W3/1(w1)
  w2/1 -> Product1/2
  Demux4/3 -> W2/3(w3)
  Demux4/2 -> W2/2(w2)
  Demux4/1 -> W2/1(w1)
  w1/1 -> Product/2
  Demux5/3 -> W1/3(w3)
  Demux5/2 -> W1/2(w2)
  Demux5/1 -> W1/1(w1)
  Product/1 -> Demux5/1
  Product1/1 -> Demux4/1
  Product2/1 -> Demux3/1
  Product3/1 -> Demux2/1
  Product4/1 -> Demux1/1
  Product5/1 -> Demux/1

== system Dynamics/DYNAMIC/Moments of inertia/Ix, Iy ==
  r : Inport
  m : Inport  Port=2
  h : Inport  Port=3
  Add : Sum
  Gain : Gain  Gain=3
  Gain1 : Gain  Gain=1/12
  Product : Product
  Product1 : Product
  Product2 : Product
  Iz : Outport
  wires:
  r/1 -> Product/1, Product/2
  h/1 -> Product1/1, Product1/2
  Product/1 -> Gain/1
  Product1/1 -> Add/2
  Add/1 -> Product2/1
  m/1 -> Product2/2
  Gain/1 -> Add/1
  Product2/1 -> Gain1/1
  Gain1/1 -> Iz/1

== system Dynamics/DYNAMIC/Moments of inertia/Ix, Iy1 ==
  r : Inport
  m : Inport  Port=2
  h : Inport  Port=3
  Add : Sum
  Gain : Gain  Gain=3
  Gain1 : Gain  Gain=1/12
  Product : Product
  Product1 : Product
  Product2 : Product
  Iz : Outport
  wires:
  r/1 -> Product/1, Product/2
  h/1 -> Product1/1, Product1/2
  Product/1 -> Gain/1
  Product1/1 -> Add/2
  Add/1 -> Product2/1
  m/1 -> Product2/2
  Gain/1 -> Add/1
  Product2/1 -> Gain1/1
  Gain1/1 -> Iz/1

== system Dynamics/DYNAMIC/Moments of inertia/Ix, Iy2 ==
  r : Inport
  m : Inport  Port=2
  h : Inport  Port=3
  Add : Sum
  Gain : Gain  Gain=3
  Gain1 : Gain  Gain=1/12
  Product : Product
  Product1 : Product
  Product2 : Product
  Iz : Outport
  wires:
  r/1 -> Product/1, Product/2
  h/1 -> Product1/1, Product1/2
  Product/1 -> Gain/1
  Product1/1 -> Add/2
  Add/1 -> Product2/1
  m/1 -> Product2/2
  Gain/1 -> Add/1
  Product2/1 -> Gain1/1
  Gain1/1 -> Iz/1

== system Dynamics/DYNAMIC/Moments of inertia/Ix, Iy3 ==
  r : Inport
  m : Inport  Port=2
  h : Inport  Port=3
  Add : Sum
  Gain : Gain  Gain=3
  Gain1 : Gain  Gain=1/12
  Product : Product
  Product1 : Product
  Product2 : Product
  Iz : Outport
  wires:
  r/1 -> Product/1, Product/2
  h/1 -> Product1/1, Product1/2
  Product/1 -> Gain/1
  Product1/1 -> Add/2
  Add/1 -> Product2/1
  m/1 -> Product2/2
  Gain/1 -> Add/1
  Product2/1 -> Gain1/1
  Gain1/1 -> Iz/1

== system Dynamics/DYNAMIC/Moments of inertia/Ix, Iy4 ==
  r : Inport
  m : Inport  Port=2
  h : Inport  Port=3
  Add : Sum
  Gain : Gain  Gain=3
  Gain1 : Gain  Gain=1/12
  Product : Product
  Product1 : Product
  Product2 : Product
  Iz : Outport
  wires:
  r/1 -> Product/1, Product/2
  h/1 -> Product1/1, Product1/2
  Product/1 -> Gain/1
  Product1/1 -> Add/2
  Add/1 -> Product2/1
  m/1 -> Product2/2
  Gain/1 -> Add/1
  Product2/1 -> Gain1/1
  Gain1/1 -> Iz/1

== system Dynamics/DYNAMIC/Moments of inertia/Ix, Iy5 ==
  r : Inport
  m : Inport  Port=2
  h : Inport  Port=3
  Add : Sum
  Gain : Gain  Gain=3
  Gain1 : Gain  Gain=1/12
  Product : Product
  Product1 : Product
  Product2 : Product
  Iz : Outport
  wires:
  r/1 -> Product/1, Product/2
  h/1 -> Product1/1, Product1/2
  Product/1 -> Gain/1
  Product1/1 -> Add/2
  Add/1 -> Product2/1
  m/1 -> Product2/2
  Gain/1 -> Add/1
  Product2/1 -> Gain1/1
  Gain1/1 -> Iz/1

== system Dynamics/DYNAMIC/Moments of inertia/Iz ==
  r : Inport
  m : Inport  Port=2
  Constant : Constant  Value=0.5
  Product : Product  Inputs=4
  Iz : Outport
  wires:
  m/1 -> Product/3
  Constant/1 -> Product/4
  r/1 -> Product/2, Product/1
  Product/1 -> Iz/1

== system Dynamics/DYNAMIC/Moments of inertia/Iz1 ==
  r : Inport
  m : Inport  Port=2
  Constant : Constant  Value=0.5
  Product : Product  Inputs=4
  Iz : Outport
  wires:
  m/1 -> Product/3
  Constant/1 -> Product/4
  r/1 -> Product/2, Product/1
  Product/1 -> Iz/1

== system Dynamics/DYNAMIC/Moments of inertia/Iz2 ==
  r : Inport
  m : Inport  Port=2
  Constant : Constant  Value=0.5
  Product : Product  Inputs=4
  Iz : Outport
  wires:
  m/1 -> Product/3
  Constant/1 -> Product/4
  r/1 -> Product/2, Product/1
  Product/1 -> Iz/1

== system Dynamics/DYNAMIC/Moments of inertia/Iz3 ==
  r : Inport
  m : Inport  Port=2
  Constant : Constant  Value=0.5
  Product : Product  Inputs=4
  Iz : Outport
  wires:
  m/1 -> Product/3
  Constant/1 -> Product/4
  r/1 -> Product/2, Product/1
  Product/1 -> Iz/1

== system Dynamics/DYNAMIC/Moments of inertia/Iz4 ==
  r : Inport
  m : Inport  Port=2
  Constant : Constant  Value=0.5
  Product : Product  Inputs=4
  Iz : Outport
  wires:
  m/1 -> Product/3
  Constant/1 -> Product/4
  r/1 -> Product/2, Product/1
  Product/1 -> Iz/1

== system Dynamics/DYNAMIC/Moments of inertia/Iz5 ==
  r : Inport
  m : Inport  Port=2
  Constant : Constant  Value=0.5
  Product : Product  Inputs=4
  Iz : Outport
  wires:
  m/1 -> Product/3
  Constant/1 -> Product/4
  r/1 -> Product/2, Product/1
  Product/1 -> Iz/1

== system Dynamics/DYNAMIC/Slotine/S-gen ==
  dq : Inport
  V : Inport  Port=2
  Gain : Gain  Gain=-1
  Sum : Sum  Inputs=|++
  S : Outport
  wires:
  dq/1 -> Sum/1
  Sum/1 -> S/1
  V/1 -> Gain/1
  Gain/1 -> Sum/2

== system Dynamics/DYNAMIC/Slotine/V-gen ==
  q_tilde : Inport
  dq_d : Inport  Port=2
  Gamma : Inport  Port=3
  Gain : Gain  Gain=-1
  Product : Product  Multiplication=Matrix(*)
  Sum : Sum  Inputs=|++
  V : Outport
  wires:
  Gamma/1 -> Product/1
  q_tilde/1 -> Product/2
  Product/1 -> Gain/1
  Sum/1 -> V/1
  dq_d/1 -> Sum/1
  Gain/1 -> Sum/2

== system Dynamics/DYNAMIC/Slotine/dV-gen ==
  dq_tilde : Inport
  ddq_d : Inport  Port=2
  Gamma : Inport  Port=3
  Gain : Gain  Gain=-1
  Product : Product  Multiplication=Matrix(*)
  Sum : Sum  Inputs=|++
  dV : Outport
  wires:
  Gamma/1 -> Product/1
  dq_tilde/1 -> Product/2
  Product/1 -> Gain/1
  Sum/1 -> dV/1
  ddq_d/1 -> Sum/1
  Gain/1 -> Sum/2

== system Dynamics/DYNAMIC/Slotine/tau-gen ==
  M : Inport
  C : Inport  Port=2
  g : Inport  Port=3
  V : Inport  Port=4
  dV : Inport  Port=5
  S : Inport  Port=6
  K : Inport  Port=7
  Product : Product  Multiplication=Matrix(*)
  Product1 : Product  Multiplication=Matrix(*)
  Product2 : Product  Multiplication=Matrix(*)
  Sum : Sum  Inputs=|++
  Sum1 : Sum  Inputs=|++
  Sum2 : Sum  Inputs=|+-
  tau : Outport
  wires:
  M/1 -> Product/1
  dV/1 -> Product/2
  C/1 -> Product1/1
  V/1 -> Product1/2
  S/1 -> Product2/2
  K/1 -> Product2/1
  Product/1 -> Sum/1
  Product1/1 -> Sum/2
  Sum/1 -> Sum1/1
  g/1 -> Sum1/2
  Product2/1 -> Sum2/2
  Sum1/1 -> Sum2/1
  Sum2/1 -> tau/1

== system Dynamics/Subsystem/Dynamics/Friction ==
  dq : Inport
  d(t) : Inport  Port=2
  Constant : Constant  Value=-10
  Constant1 : Constant  Value=2
  Constant2 : Constant  Value=0
  Demux : Demux  Outputs=6
  Mux : Mux  Inputs=6
  Product : Product
  Product1 : Product
  Sign : Signum
  Sum : Sum  Inputs=|++
  Sum1 : Sum  Inputs=|++
  Sum2 : Sum  Inputs=|++
  Terminator{,1..4} (5 alike) : Terminator
  tau_f : Outport
  wires:
  dq/1 -> Demux/1
  Demux/6 -> Terminator/1
  Demux/5 -> Terminator1/1
  Demux/4 -> Terminator2/1
  Demux/1 -> Terminator3/1
  Demux/3 -> Terminator4/1
  Demux/2 -> Sign/1, Product/1
  d(t)/1 -> Sum2/1, Sum/1
  Constant/1 -> Sum/2
  Sum/1 -> Product/2
  Product/1 -> Sum1/1
  Sum2/1 -> Product1/2
  Constant1/1 -> Sum2/2
  Sign/1 -> Product1/1
  Product1/1 -> Sum1/2
  Sum1/1 -> Mux/2
  Mux/1 -> tau_f/1
  Constant2/1 -> Mux/6, Mux/5, Mux/4, Mux/3, Mux/1

== system Dynamics/Subsystem/H_6^0/H_1^0 ==
  a : Inport
  alpha : Inport  Port=2
  theta : Inport  Port=3
  d : Inport  Port=4
  Gain1 : Gain  Gain=-1
  Gain2 : Gain  Gain=-1
  MATLAB Function : MATLAB Function  TreatAsAtomicUnit=on
  Mux : Mux  Inputs=3
  Mux1 : Mux  Inputs=3
  Product : Product
  Product1 : Product
  Rotation Angles to Direction Cosine Matrix : sharedtransform/Rotation Angles to Direction Cosine Matrix  rotationOrder=ZXY  aMode=aMode
  Trigonometric Function : Trigonometry  Operator=cos
  Trigonometric Function1 : Trigonometry
  Zero : Constant  Value=0
  H : Outport
  R : Outport  Port=2
  p : Outport  Port=3
  wires:
  Mux/1 -> Rotation Angles to Direction Cosine Matrix/1
  alpha/1 -> Gain1/1
  Zero/1 -> Mux/3
  Rotation Angles to Direction Cosine Matrix/1 -> MATLAB Function/1(R), R/1
  Mux1/1 -> MATLAB Function/2(p), p/1
  Trigonometric Function/1 -> Product/1
  Trigonometric Function1/1 -> Product1/1
  Product/1 -> Mux1/1
  Product1/1 -> Mux1/2
  a/1 -> Product/2, Product1/2
  MATLAB Function/1(H) -> H/1
  Gain1/1 -> Mux/1
  Gain2/1 -> Mux/2
  theta/1 -> Trigonometric Function1/1, Trigonometric Function/1, Gain2/1
  d/1 -> Mux1/3

== system Dynamics/Subsystem/H_6^0/H_2^1 ==
  a : Inport
  alpha : Inport  Port=2
  theta : Inport  Port=3
  d : Inport  Port=4
  Gain1 : Gain  Gain=-1
  Gain2 : Gain  Gain=-1
  MATLAB Function : MATLAB Function  TreatAsAtomicUnit=on
  Mux : Mux  Inputs=3
  Mux1 : Mux  Inputs=3
  Product : Product
  Product1 : Product
  Rotation Angles to Direction Cosine Matrix : sharedtransform/Rotation Angles to Direction Cosine Matrix  rotationOrder=ZXY  aMode=aMode
  Trigonometric Function : Trigonometry  Operator=cos
  Trigonometric Function1 : Trigonometry
  Zero : Constant  Value=0
  H : Outport
  R : Outport  Port=2
  p : Outport  Port=3
  wires:
  Mux/1 -> Rotation Angles to Direction Cosine Matrix/1
  alpha/1 -> Gain1/1
  Zero/1 -> Mux/3
  Rotation Angles to Direction Cosine Matrix/1 -> MATLAB Function/1(R), R/1
  Mux1/1 -> MATLAB Function/2(p), p/1
  Trigonometric Function/1 -> Product/1
  Trigonometric Function1/1 -> Product1/1
  Product/1 -> Mux1/1
  Product1/1 -> Mux1/2
  a/1 -> Product/2, Product1/2
  MATLAB Function/1(H) -> H/1
  Gain1/1 -> Mux/1
  Gain2/1 -> Mux/2
  theta/1 -> Trigonometric Function1/1, Trigonometric Function/1, Gain2/1
  d/1 -> Mux1/3

== system Dynamics/Subsystem/H_6^0/H_3^2 ==
  a : Inport
  alpha : Inport  Port=2
  theta : Inport  Port=3
  d : Inport  Port=4
  Gain1 : Gain  Gain=-1
  Gain2 : Gain  Gain=-1
  MATLAB Function : MATLAB Function  TreatAsAtomicUnit=on
  Mux : Mux  Inputs=3
  Mux1 : Mux  Inputs=3
  Product : Product
  Product1 : Product
  Rotation Angles to Direction Cosine Matrix : sharedtransform/Rotation Angles to Direction Cosine Matrix  rotationOrder=ZXY  aMode=aMode
  Trigonometric Function : Trigonometry  Operator=cos
  Trigonometric Function1 : Trigonometry
  Zero : Constant  Value=0
  H : Outport
  R : Outport  Port=2
  p : Outport  Port=3
  wires:
  Mux/1 -> Rotation Angles to Direction Cosine Matrix/1
  alpha/1 -> Gain1/1
  Zero/1 -> Mux/3
  Rotation Angles to Direction Cosine Matrix/1 -> MATLAB Function/1(R), R/1
  Mux1/1 -> MATLAB Function/2(p), p/1
  Trigonometric Function/1 -> Product/1
  Trigonometric Function1/1 -> Product1/1
  Product/1 -> Mux1/1
  Product1/1 -> Mux1/2
  a/1 -> Product/2, Product1/2
  MATLAB Function/1(H) -> H/1
  Gain1/1 -> Mux/1
  Gain2/1 -> Mux/2
  theta/1 -> Trigonometric Function1/1, Trigonometric Function/1, Gain2/1
  d/1 -> Mux1/3

== system Dynamics/Subsystem/H_6^0/H_4^3 ==
  a : Inport
  alpha : Inport  Port=2
  theta : Inport  Port=3
  d : Inport  Port=4
  Gain1 : Gain  Gain=-1
  Gain2 : Gain  Gain=-1
  MATLAB Function : MATLAB Function  TreatAsAtomicUnit=on
  Mux : Mux  Inputs=3
  Mux1 : Mux  Inputs=3
  Product : Product
  Product1 : Product
  Rotation Angles to Direction Cosine Matrix : sharedtransform/Rotation Angles to Direction Cosine Matrix  rotationOrder=ZXY  aMode=aMode
  Trigonometric Function : Trigonometry  Operator=cos
  Trigonometric Function1 : Trigonometry
  Zero : Constant  Value=0
  H : Outport
  R : Outport  Port=2
  p : Outport  Port=3
  wires:
  Mux/1 -> Rotation Angles to Direction Cosine Matrix/1
  alpha/1 -> Gain1/1
  Zero/1 -> Mux/3
  Rotation Angles to Direction Cosine Matrix/1 -> MATLAB Function/1(R), R/1
  Mux1/1 -> MATLAB Function/2(p), p/1
  Trigonometric Function/1 -> Product/1
  Trigonometric Function1/1 -> Product1/1
  Product/1 -> Mux1/1
  Product1/1 -> Mux1/2
  a/1 -> Product/2, Product1/2
  MATLAB Function/1(H) -> H/1
  Gain1/1 -> Mux/1
  Gain2/1 -> Mux/2
  theta/1 -> Trigonometric Function1/1, Trigonometric Function/1, Gain2/1
  d/1 -> Mux1/3

== system Dynamics/Subsystem/H_6^0/H_5^4 ==
  a : Inport
  alpha : Inport  Port=2
  theta : Inport  Port=3
  d : Inport  Port=4
  Gain1 : Gain  Gain=-1
  Gain2 : Gain  Gain=-1
  MATLAB Function : MATLAB Function  TreatAsAtomicUnit=on
  Mux : Mux  Inputs=3
  Mux1 : Mux  Inputs=3
  Product : Product
  Product1 : Product
  Rotation Angles to Direction Cosine Matrix : sharedtransform/Rotation Angles to Direction Cosine Matrix  rotationOrder=ZXY  aMode=aMode
  Trigonometric Function : Trigonometry  Operator=cos
  Trigonometric Function1 : Trigonometry
  Zero : Constant  Value=0
  H : Outport
  R : Outport  Port=2
  p : Outport  Port=3
  wires:
  Mux/1 -> Rotation Angles to Direction Cosine Matrix/1
  alpha/1 -> Gain1/1
  Zero/1 -> Mux/3
  Rotation Angles to Direction Cosine Matrix/1 -> MATLAB Function/1(R), R/1
  Mux1/1 -> MATLAB Function/2(p), p/1
  Trigonometric Function/1 -> Product/1
  Trigonometric Function1/1 -> Product1/1
  Product/1 -> Mux1/1
  Product1/1 -> Mux1/2
  a/1 -> Product/2, Product1/2
  MATLAB Function/1(H) -> H/1
  Gain1/1 -> Mux/1
  Gain2/1 -> Mux/2
  theta/1 -> Trigonometric Function1/1, Trigonometric Function/1, Gain2/1
  d/1 -> Mux1/3

== system Dynamics/Subsystem/H_6^0/H_6^5 ==
  a : Inport
  alpha : Inport  Port=2
  theta : Inport  Port=3
  d : Inport  Port=4
  Gain1 : Gain  Gain=-1
  Gain2 : Gain  Gain=-1
  MATLAB Function : MATLAB Function  TreatAsAtomicUnit=on
  Mux : Mux  Inputs=3
  Mux1 : Mux  Inputs=3
  Product : Product
  Product1 : Product
  Rotation Angles to Direction Cosine Matrix : sharedtransform/Rotation Angles to Direction Cosine Matrix  rotationOrder=ZXY  aMode=aMode
  Trigonometric Function : Trigonometry  Operator=cos
  Trigonometric Function1 : Trigonometry
  Zero : Constant  Value=0
  H : Outport
  R : Outport  Port=2
  p : Outport  Port=3
  wires:
  Mux/1 -> Rotation Angles to Direction Cosine Matrix/1
  alpha/1 -> Gain1/1
  Zero/1 -> Mux/3
  Rotation Angles to Direction Cosine Matrix/1 -> MATLAB Function/1(R), R/1
  Mux1/1 -> MATLAB Function/2(p), p/1
  Trigonometric Function/1 -> Product/1
  Trigonometric Function1/1 -> Product1/1
  Product/1 -> Mux1/1
  Product1/1 -> Mux1/2
  a/1 -> Product/2, Product1/2
  MATLAB Function/1(H) -> H/1
  Gain1/1 -> Mux/1
  Gain2/1 -> Mux/2
  theta/1 -> Trigonometric Function1/1, Trigonometric Function/1, Gain2/1
  d/1 -> Mux1/3

== system Dynamics/Subsystem/Jacobian/J(q) gen. ==
  R_1^0 : Inport
  R_2^0 : Inport  Port=2
  R_3^0 : Inport  Port=3
  R_4^0 : Inport  Port=4
  R_5^0 : Inport  Port=5
  R_6^0 : Inport  Port=6
  p_1^0 : Inport  Port=7
  p_2^0 : Inport  Port=8
  p_3^0 : Inport  Port=9
  p_4^0 : Inport  Port=10
  p_5^0 : Inport  Port=11
  type1 : Inport  Port=12
  type2 : Inport  Port=13
  type3 : Inport  Port=14
  type4 : Inport  Port=15
  J_v_6(q) : Inport  Port=16
  J_w1 : Inport  Port=17
  J_w2 : Inport  Port=18
  J_w3 : Inport  Port=19
  J_w4 : Inport  Port=20
  J_w5 : Inport  Port=21
  J_w6 : Inport  Port=22
  J_v_1(q) : Subsystem
  J_v_2(q) : Subsystem
  J_v_3(q) : Subsystem
  J_v_4(q) : Subsystem
  J_v_5(q) : Subsystem
  MATLAB Function : MATLAB Function  TreatAsAtomicUnit=on
  J(q) : Outport
  wires:
  MATLAB Function/1(J_q) -> J(q)/1
  J_v_6(q)/1 -> MATLAB Function/12(J_v6)
  J_w1/1 -> MATLAB Function/1(J_w1)
  J_w2/1 -> MATLAB Function/2(J_w2)
  J_w3/1 -> MATLAB Function/3(J_w3)
  J_w4/1 -> MATLAB Function/4(J_w4)
  J_w5/1 -> MATLAB Function/5(J_w5)
  J_w6/1 -> MATLAB Function/6(J_w6)
  J_v_1(q)/1(J_v_1(q)) -> MATLAB Function/7(J_v1)
  J_v_2(q)/1(J_v_2(q)) -> MATLAB Function/8(J_v2)
  J_v_3(q)/1(J_v_3(q)) -> MATLAB Function/9(J_v3)
  J_v_4(q)/1(J_v_4(q)) -> MATLAB Function/10(J_v4)
  J_v_5(q)/1(J_v_5(q)) -> MATLAB Function/11(J_v5)
  R_5^0/1 -> MATLAB Function/17(R5)
  R_6^0/1 -> MATLAB Function/18(R6)
  R_1^0/1 -> MATLAB Function/13(R1), J_v_5(q)/1(R_1^0), J_v_4(q)/1(R_1^0), J_v_3(q)/1(R_1^0), J_v_2(q)/1(R_1^0)
  R_2^0/1 -> MATLAB Function/14(R2), J_v_5(q)/2(R_2^0), J_v_4(q)/2(R_2^0), J_v_3(q)/2(R_2^0)
  R_3^0/1 -> J_v_4(q)/3(R_3^0), MATLAB Function/15(R3), J_v_5(q)/3(R_3^0)
  R_4^0/1 -> MATLAB Function/16(R4), J_v_5(q)/4(R_4^0)
  p_1^0/1 -> J_v_5(q)/5(p_1^0), J_v_4(q)/4(p_1^0), J_v_3(q)/3(p_1^0), J_v_2(q)/2(p_1^0)
  p_2^0/1 -> J_v_5(q)/6(p_2^0), J_v_4(q)/5(p_2^0), J_v_3(q)/4(p_2^0), J_v_2(q)/3(p_2^0)
  p_3^0/1 -> J_v_3(q)/5(p_3^0), J_v_5(q)/7(p_3^0), J_v_4(q)/6(p_3^0)
  p_4^0/1 -> J_v_5(q)/8(p_4^0), J_v_4(q)/7(p_4^0)
  p_5^0/1 -> J_v_5(q)/9(p_5^0)
  type1/1 -> J_v_5(q)/10(type1), J_v_4(q)/8(type1), J_v_3(q)/6(type1), J_v_2(q)/4(type1)
  type2/1 -> J_v_5(q)/11(type2), J_v_4(q)/9(type2), J_v_3(q)/7(type2)
  type3/1 -> J_v_5(q)/12(type3), J_v_4(q)/10(type3)
  type4/1 -> J_v_5(q)/13(type4)

== system Dynamics/Subsystem/Jacobian/J_v ==
  R_1^0 : Inport
  R_2^0 : Inport  Port=2
  R_3^0 : Inport  Port=3
  R_4^0 : Inport  Port=4
  R_5^0 : Inport  Port=5
  R_6^0 : Inport  Port=6
  p_1^0 : Inport  Port=7
  p_2^0 : Inport  Port=8
  p_3^0 : Inport  Port=9
  p_4^0 : Inport  Port=10
  p_5^0 : Inport  Port=11
  p_6^0 : Inport  Port=12
  type1 : Inport  Port=13
  type2 : Inport  Port=14
  type3 : Inport  Port=15
  type4 : Inport  Port=16
  type5 : Inport  Port=17
  type6 : Inport  Port=18
  J_v_1 : Subsystem
  J_v_2 : Subsystem
  J_v_3 : Subsystem
  J_v_4 : Subsystem
  J_v_5 : Subsystem
  J_v_6 : Subsystem
  v2M_1 : MATLAB Function  TreatAsAtomicUnit=on
  v2M_2 : MATLAB Function  TreatAsAtomicUnit=on
  v2M_3 : MATLAB Function  TreatAsAtomicUnit=on
  v2M_4 : MATLAB Function  TreatAsAtomicUnit=on
  v2M_5 : MATLAB Function  TreatAsAtomicUnit=on
  J_v : Outport
  wires:
  R_1^0/1 -> J_v_1/1(R)
  J_v_1/1(J_v) -> v2M_1/1(v1)
  v2M_1/1(M) -> v2M_2/1(v1)
  v2M_2/1(M) -> v2M_3/1(v1)
  v2M_3/1(M) -> v2M_4/1(v1)
  v2M_4/1(M) -> v2M_5/1(v1)
  v2M_5/1(M) -> J_v/1
  J_v_2/1(J_v) -> v2M_1/2(v2)
  J_v_3/1(J_v) -> v2M_2/2(v2)
  J_v_4/1(J_v) -> v2M_3/2(v2)
  J_v_5/1(J_v) -> v2M_4/2(v2)
  J_v_6/1(J_v) -> v2M_5/2(v2)
  R_2^0/1 -> J_v_2/1(R)
  R_3^0/1 -> J_v_3/1(R)
  R_4^0/1 -> J_v_4/1(R)
  R_5^0/1 -> J_v_5/1(R)
  R_6^0/1 -> J_v_6/1(R)
  p_1^0/1 -> J_v_1/2(p)
  p_2^0/1 -> J_v_2/2(p)
  p_3^0/1 -> J_v_3/2(p)
  p_4^0/1 -> J_v_4/2(p)
  p_5^0/1 -> J_v_5/2(p)
  type2/1 -> J_v_2/4(type)
  type1/1 -> J_v_1/4(type)
  type3/1 -> J_v_3/4(type)
  type4/1 -> J_v_4/4(type)
  type5/1 -> J_v_5/4(type)
  type6/1 -> J_v_6/4(type)
  p_6^0/1 -> J_v_6/2(p), J_v_1/3(pn), J_v_2/3(pn), J_v_3/3(pn), J_v_4/3(pn), J_v_5/3(pn), J_v_6/3(pn)

== system Dynamics/Subsystem/Jacobian/J_w ==
  R_1^0 : Inport
  R_2^0 : Inport  Port=2
  R_3^0 : Inport  Port=3
  R_4^0 : Inport  Port=4
  R_5^0 : Inport  Port=5
  R_6^0 : Inport  Port=6
  type1 : Inport  Port=7
  type2 : Inport  Port=8
  type3 : Inport  Port=9
  type4 : Inport  Port=10
  type5 : Inport  Port=11
  type6 : Inport  Port=12
  J_w_1 : MATLAB Function  TreatAsAtomicUnit=on
  J_w_2 : MATLAB Function  TreatAsAtomicUnit=on
  J_w_3 : MATLAB Function  TreatAsAtomicUnit=on
  J_w_4 : MATLAB Function  TreatAsAtomicUnit=on
  J_w_5 : MATLAB Function  TreatAsAtomicUnit=on
  J_w_6 : MATLAB Function  TreatAsAtomicUnit=on
  v2M_1 : MATLAB Function  TreatAsAtomicUnit=on
  v2M_2 : MATLAB Function  TreatAsAtomicUnit=on
  v2M_3 : MATLAB Function  TreatAsAtomicUnit=on
  v2M_4 : MATLAB Function  TreatAsAtomicUnit=on
  v2M_5 : MATLAB Function  TreatAsAtomicUnit=on
  EF J_w : Outport
  J_w1 : Outport  Port=2
  J_w2 : Outport  Port=3
  J_w3 : Outport  Port=4
  J_w4 : Outport  Port=5
  J_w5 : Outport  Port=6
  J_w6 : Outport  Port=7
  wires:
  R_1^0/1 -> J_w_1/1(R)
  R_2^0/1 -> J_w_2/1(R)
  R_3^0/1 -> J_w_3/1(R)
  R_4^0/1 -> J_w_4/1(R)
  R_5^0/1 -> J_w_5/1(R)
  R_6^0/1 -> J_w_6/1(R)
  J_w_1/1(J_w) -> J_w1/1, v2M_1/1(v1)
  J_w_2/1(J_w) -> J_w2/1, v2M_1/2(v2)
  J_w_3/1(J_w) -> J_w3/1, v2M_2/2(v2)
  v2M_1/1(M) -> v2M_2/1(v1)
  v2M_2/1(M) -> v2M_3/1(v1)
  v2M_3/1(M) -> v2M_4/1(v1)
  J_w_5/1(J_w) -> J_w5/1, v2M_4/2(v2)
  J_w_6/1(J_w) -> J_w6/1, v2M_5/2(v2)
  v2M_4/1(M) -> v2M_5/1(v1)
  v2M_5/1(M) -> EF J_w/1
  type1/1 -> J_w_1/2(type)
  type2/1 -> J_w_2/2(type)
  type3/1 -> J_w_3/2(type)
  type4/1 -> J_w_4/2(type)
  type5/1 -> J_w_5/2(type)
  type6/1 -> J_w_6/2(type)
  J_w_4/1(J_w) -> v2M_3/2(v2), J_w4/1
